simulink model "TAU_Khomutov_11_model"  (R2014a)
settings: Solver=VariableStepAuto  StartTime=0.0  StopTime=10.0  RelTol=1e-3
values from neighbouring files (symbols this model uses):
  a = [1 21.2 26.247 7.217 1.601 0.376]    [TAU_Khomutov_11_script.m]
  Amplitude = 1.57 * 10 ^ (-6)    (= 1.57e-06)    [TAU_Khomutov_11_script.m]
  b = [1.25 1.626 0.376]    [TAU_Khomutov_11_script.m]
  E = eye(rA)    [TAU_Khomutov_11_script.m]
  K = acker (A,B,Pc)    [TAU_Khomutov_11_script.m]
  L = acker(A',C',P0)'    [TAU_Khomutov_11_script.m]
  rA = rank (A)    [TAU_Khomutov_11_script.m]
undefined symbols (not defined in the file or in its folder): A, B, C
settings Model: Creator=sergey  LastModifiedBy=Evgeny
settings DataIOCC: LimitDataPoints=off  SaveFormat=Dataset
settings OptimizationCC: LifeSpan=auto  SimCompilerOptimization=off
settings DebuggingCC: MergeDetectMultiDrivingBlocksExec=error  SolverPrmCheckMsg=none  FcnCallInpInsideContextMsg=error  FrameProcessingCompatibilityMsg=error  SFUnexpectedBacktrackingDiag=error  SFNoUnconditionalDefaultTransitionDiag=error
settings HardwareCC: ProdBitPerPointer=64  ProdLargestAtomicFloat=Float  ProdIntDivRoundTo=Zero  ProdEndianess=LittleEndian  ProdWordSize=64  ProdHWDeviceType=Intel->x86-64 (Windows64)
settings ModelReferenceCC: PropagateSignalLabelsOutOfModel=on
settings RTWCC: RTWCompilerOptimization=off
settings GRTTargetCC: TargetLangStandard=C99 (ISO)  GeneratePreprocessorConditionals=Use local settings

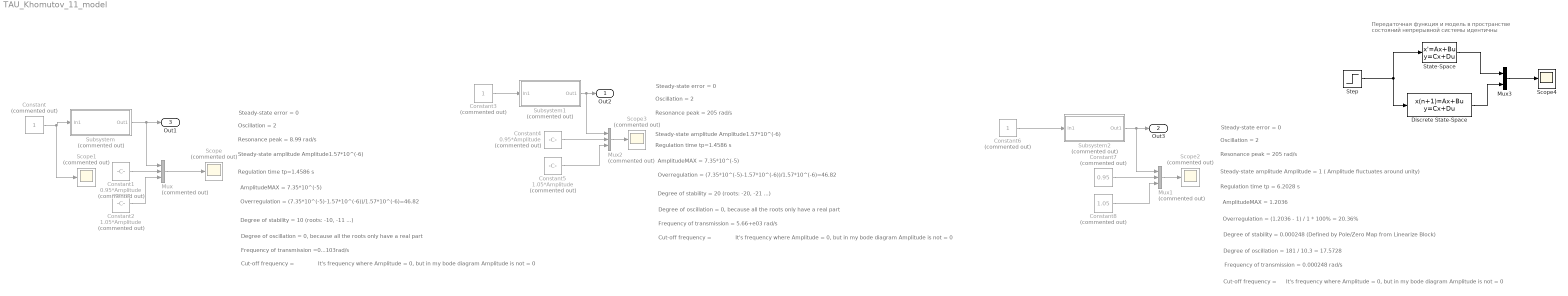
== system TAU_Khomutov_11_model ==
  note: Передаточная функция и модель в пространстве
      | состояний непрерывной системы идентичны
  note: It's frequency where Amplitude = 0, but in my bode diagram Amplitude is not = 0
  note: Cut-off frequency =
  note: Frequency of transmission =0...103rad/s
  note: Degree of oscillation = 0, because all the roots only have a real part
  note: Degree of stability = 10 (roots: -10, -11 ...)
  note: Steady-state error = 0
  note: Oscillation = 2
  note: Overregulation = (7.35*10^(-5)-1.57*10^(-6))/1.57*10^(-6)=46.82
  note: AmplitudeMAX = 7.35*10^(-5)
  note: Regulation time tp=1.4586 s
  note: Steady-state amplitude Amplitude1.57*10^(-6)
  note: Resonance peak = 8.99 rad/s
  note: It's frequency where Amplitude = 0, but in my bode diagram Amplitude is not = 0
  note: Cut-off frequency =
  note: Frequency of transmission = 5.66+e03 rad/s
  note: Degree of oscillation = 0, because all the roots only have a real part
  note: Degree of stability = 20 (roots: -20, -21 ...)
  note: Steady-state error = 0
  note: Oscillation = 2
  note: Overregulation = (7.35*10^(-5)-1.57*10^(-6))/1.57*10^(-6)=46.82
  note: AmplitudeMAX = 7.35*10^(-5)
  note: Regulation time tp=1.4586 s
  note: Steady-state amplitude Amplitude1.57*10^(-6)
  note: Resonance peak = 205 rad/s
  note: It's frequency where Amplitude = 0, but in my bode diagram Amplitude is not = 0
  note: Cut-off frequency =
  note: Frequency of transmission = 0.000248 rad/s
  note: Degree of oscillation = 181 / 10.3 = 17.5728
  note: Degree of stability = 0.000248 (Defined by Pole/Zero Map from Linearize Block)
  note: Steady-state error = 0
  note: Oscillation = 2
  note: Overregulation = (1.2036 - 1) / 1 * 100% = 20.36%
  note: AmplitudeMAX = 1.2036
  note: Regulation time tp = 6.2028 s
  note: Steady-state amplitude Amplitude = 1 ( Amplitude fluctuates around unity)
  note: Resonance peak = 205 rad/s
  Constant : Constant  Commented=on
  Constant1 : Constant  Commented=on  Value=0.95*Amplitude
  Constant2 : Constant  Commented=on  Value=1.05*Amplitude
  Constant3 : Constant  Commented=on
  Constant4 : Constant  Commented=on  Value=0.95*Amplitude
  Constant5 : Constant  Commented=on  Value=1.05*Amplitude
  Constant6 : Constant  Commented=on
  Constant7 : Constant  Commented=on  Value=0.95
  Constant8 : Constant  Commented=on  Value=1.05
  Discrete State-Space : DiscreteStateSpace  A=eye(5)+A*0.001  B=B*0.001  C=C  D=0  SampleTime=0.001
  Mux : Mux  Commented=on  Inputs=3
  Mux1 : Mux  Commented=on  Inputs=3
  Mux2 : Mux  Commented=on  Inputs=3
  Mux3 : Mux  Inputs=2
  Scope{,1..3} (4 alike) : Scope  Commented=on
      Scope settings: TimeRange=6.71088640000761e-05  YMin=1.490725903150069e-06  YMax=1.491531209518069e-06
      Scope1 settings: TimeRange=6.71088640000761e-05  YMin=1.490725903150069e-06  YMax=1.491531209518069e-06
      Scope2 settings: TimeRange=2.801837117871742e-07  YMin=1.574574372556849e-06  YMax=1.574612058926273e-06  SaveName=ScopeData2
      Scope3 settings: TimeRange=6.71088640000761e-05  YMin=1.490725903150069e-06  YMax=1.491531209518069e-06  SaveName=ScopeData3
  Scope4 : Scope
      settings: SaveName=ScopeData4
  State-Space : StateSpace  A=A  B=B  C=C  D=0  X0=0
  Step : Step  SampleTime=0
  Subsystem : Subsystem  Commented=on
  Subsystem1 : Subsystem  Commented=on
  Subsystem2 : Subsystem  Commented=on
  Out2 : Outport
  Out3 : Outport  Port=2
  Out1 : Outport  Port=3
  wires:
  Constant1/1 -> Mux/2
  Constant2/1 -> Mux/3
  Mux/1 -> Scope/1
  Constant/1 -> Subsystem/1(In1), Scope1/1
  Constant4/1 -> Mux2/2
  Constant5/1 -> Mux2/3
  Mux2/1 -> Scope3/1
  Constant7/1 -> Mux1/2
  Constant8/1 -> Mux1/3
  Mux1/1 -> Scope2/1
  Mux3/1 -> Scope4/1
  Step/1 -> Discrete State-Space/1, State-Space/1
  Subsystem/1(Out1) -> Mux/1, Out1/1
  Constant3/1 -> Subsystem1/1(In1)
  Subsystem1/1(Out1) -> Mux2/1, Out2/1
  Subsystem2/1(Out1) -> Mux1/1, Out3/1
  Constant6/1 -> Subsystem2/1(In1)
  Discrete State-Space/1 -> Mux3/2
  State-Space/1 -> Mux3/1

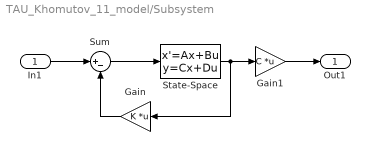
== system TAU_Khomutov_11_model/Subsystem ==
  In1 : Inport
  Gain : Gain  Gain=K  Multiplication=Matrix(K*u)
  Gain1 : Gain  Gain=C  Multiplication=Matrix(K*u)
  State-Space : StateSpace  A=A  B=B  C=E  D=zeros(rA,1)  X0=0
  Sum : Sum  Inputs=|+-
  Out1 : Outport
  wires:
  Sum/1 -> State-Space/1
  In1/1 -> Sum/1
  State-Space/1 -> Gain1/1, Gain/1
  Gain/1 -> Sum/2
  Gain1/1 -> Out1/1

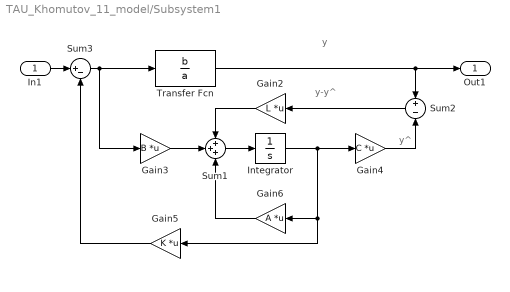
== system TAU_Khomutov_11_model/Subsystem1 ==
  note: y^
  note: y-y^
  note: y
  In1 : Inport
  Gain2 : Gain  Gain=L  Multiplication=Matrix(K*u)
  Gain3 : Gain  Gain=B  Multiplication=Matrix(K*u)
  Gain4 : Gain  Gain=C  Multiplication=Matrix(K*u)
  Gain5 : Gain  Gain=K  Multiplication=Matrix(K*u)
  Gain6 : Gain  Gain=A  Multiplication=Matrix(K*u)
  Integrator : Integrator
  Sum1 : Sum  Inputs=+++
  Sum2 : Sum  Inputs=+-
  Sum3 : Sum  Inputs=|+-
  Transfer Fcn : TransferFcn  Numerator=b  Denominator=a
  Out1 : Outport
  wires:
  Gain3/1 -> Sum1/2
  Gain6/1 -> Sum1/3
  Sum1/1 -> Integrator/1
  Integrator/1 -> Gain5/1, Gain6/1, Gain4/1
  Gain4/1 -> Sum2/2
  Sum2/1 -> Gain2/1
  Gain2/1 -> Sum1/1
  Gain5/1 -> Sum3/2
  Sum3/1 -> Gain3/1, Transfer Fcn/1
  Transfer Fcn/1 -> Out1/1, Sum2/1
  In1/1 -> Sum3/1

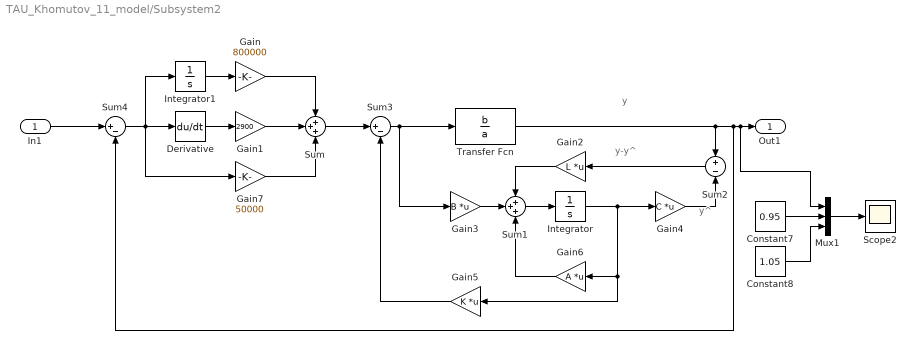
== system TAU_Khomutov_11_model/Subsystem2 ==
  note: y^
  note: y-y^
  note: y
  In1 : Inport
  Constant7 : Constant  Value=0.95
  Constant8 : Constant  Value=1.05
  Derivative : Derivative
  Gain : Gain  Gain=800000
  Gain1 : Gain  Gain=2900
  Gain2 : Gain  Gain=L  Multiplication=Matrix(K*u)
  Gain3 : Gain  Gain=B  Multiplication=Matrix(K*u)
  Gain4 : Gain  Gain=C  Multiplication=Matrix(K*u)
  Gain5 : Gain  Gain=K  Multiplication=Matrix(K*u)
  Gain6 : Gain  Gain=A  Multiplication=Matrix(K*u)
  Gain7 : Gain  Gain=50000
  Integrator : Integrator
  Integrator1 : Integrator
  Mux1 : Mux  Inputs=3
  Scope2 : Scope
      settings: TimeRange=2.801837117871742e-07  YMin=1.574574372556849e-06  YMax=1.574612058926273e-06  SaveName=ScopeData5
  Sum : Sum  Inputs=+++
  Sum1 : Sum  Inputs=+++
  Sum2 : Sum  Inputs=+-
  Sum3 : Sum  Inputs=|+-
  Sum4 : Sum  Inputs=|+-
  Transfer Fcn : TransferFcn  Numerator=b  Denominator=a
  Out1 : Outport
  wires:
  Gain3/1 -> Sum1/2
  Gain6/1 -> Sum1/3
  Sum1/1 -> Integrator/1
  Integrator/1 -> Gain5/1, Gain6/1, Gain4/1
  Gain4/1 -> Sum2/2
  Sum2/1 -> Gain2/1
  Gain2/1 -> Sum1/1
  Gain5/1 -> Sum3/2
  Sum3/1 -> Gain3/1, Transfer Fcn/1
  Transfer Fcn/1 -> Sum4/2, Mux1/1, Out1/1, Sum2/1
  In1/1 -> Sum4/1
  Sum4/1 -> Integrator1/1, Derivative/1, Gain7/1
  Derivative/1 -> Gain1/1
  Gain1/1 -> Sum/2
  Sum/1 -> Sum3/1
  Gain/1 -> Sum/1
  Gain7/1 -> Sum/3
  Integrator1/1 -> Gain/1
  Constant7/1 -> Mux1/2
  Constant8/1 -> Mux1/3
  Mux1/1 -> Scope2/1
